simulink model "MBD_Triggerd_Subsystem"  (R2021b)
settings: Solver=FixedStepDiscrete  StartTime=0.0  StopTime=10.0  FixedStep=0.001  RelTol=1e-3
libraries: simulink x1
settings Model: Creator=waleed.elshemy  LastModifiedBy=waleed.elshemy
settings OptimizationCC: DefaultParameterBehavior=Inlined  UseDivisionForNetSlopeComputation=on  GainParamInheritBuiltInType=on  UseFloatMulNetSlope=on  InlineInvariantSignals=on  PassReuseOutputArgsAs=Individual arguments  ZeroExternalMemoryAtStartup=off  ZeroInternalMemoryAtStartup=off  NoFixptDivByZeroProtection=on  EfficientFloat2IntCast=on  LifeSpan=1  OptimizeBlockOrder=speed  DifferentSizesBufferReuse=on  EfficientTunableParamExpr=on
settings DebuggingCC: ParameterTunabilityLossMsg=error
settings HardwareCC: ProdLongLongMode=on
settings SFSimCC: MATLABDynamicMemAlloc=off
settings RTWCC: Description=Embedded Coder  SystemTargetFile=ert.tlc  TemplateMakefile=ert_default_tmf
settings CodeAppCC: ForceParamTrailComments=on  IgnoreCustomStorageClasses=off  OperatorAnnotations=on  SimulinkDataObjDesc=on  SFDataObjDesc=on  CustomSymbolStrGlobalVar=rt$N$M  CustomSymbolStrType=$N$M  CustomSymbolStrFcn=$N$M$F  CustomSymbolStrMacro=$N$M  InsertBlockDesc=on
settings ERTTargetCC: TargetLangStandard=C99 (ISO)  GenerateSampleERTMain=on  IncludeMdlTerminateFcn=off  CombineSignalStateStructs=on  CodeInterfacePackaging=Reusable function  SupportComplex=off  InlinedParameterPlacement=NonHierarchical  ERTCustomFileTemplate=example_file_process.tlc  ERTFilePackagingFormat=CompactWithDataFile

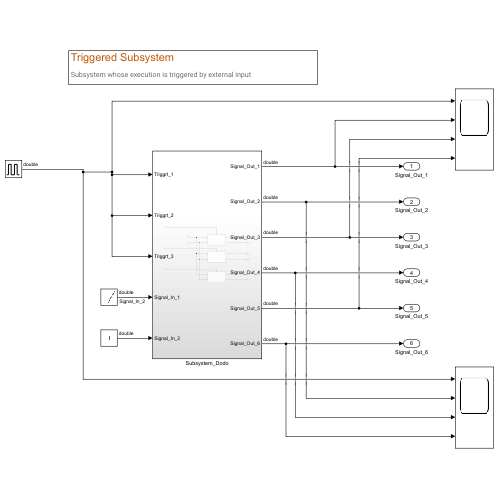
[thumbnail: Simulink's stored preview of the top-level diagram]
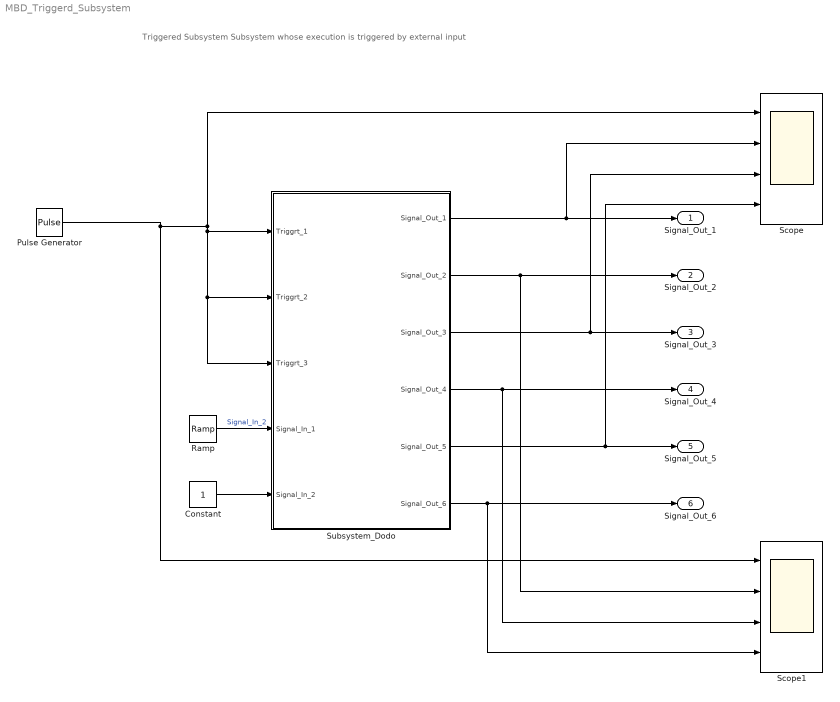
== system MBD_Triggerd_Subsystem ==
  note: Triggered Subsystem
      | Subsystem whose execution is triggered by external input
  Constant : Constant
  Pulse Generator : DiscretePulseGenerator  PulseType=Time based  Period=5  PulseWidth=50
  Ramp : simulink/Sources/Ramp  slope=1  start=0  InitialOutput=0
  Scope : Scope  NumInputPorts=4
  Scope1 : Scope  NumInputPorts=4
  Subsystem_Dodo : Subsystem
  Signal_Out_1 : Outport
  Signal_Out_2 : Outport  Port=2
  Signal_Out_3 : Outport  Port=3
  Signal_Out_4 : Outport  Port=4
  Signal_Out_5 : Outport  Port=5
  Signal_Out_6 : Outport  Port=6
  wires:
  Subsystem_Dodo/1(Signal_Out_1) -> Signal_Out_1/1, Scope/2
  Subsystem_Dodo/2(Signal_Out_2) -> Signal_Out_2/1, Scope1/2
  Subsystem_Dodo/3(Signal_Out_3) -> Signal_Out_3/1, Scope/3
  Subsystem_Dodo/4(Signal_Out_4) -> Signal_Out_4/1, Scope1/3
  Ramp/1 -> Subsystem_Dodo/4(Signal_In_1)  "Signal_In_2"
  Constant/1 -> Subsystem_Dodo/5(Signal_In_2)
  Pulse Generator/1 -> Scope1/1, Scope/1, Subsystem_Dodo/3(Triggrt_3), Subsystem_Dodo/2(Triggrt_2), Subsystem_Dodo/1(Triggrt_1)
  Subsystem_Dodo/6(Signal_Out_6) -> Signal_Out_6/1, Scope1/4
  Subsystem_Dodo/5(Signal_Out_5) -> Signal_Out_5/1, Scope/4

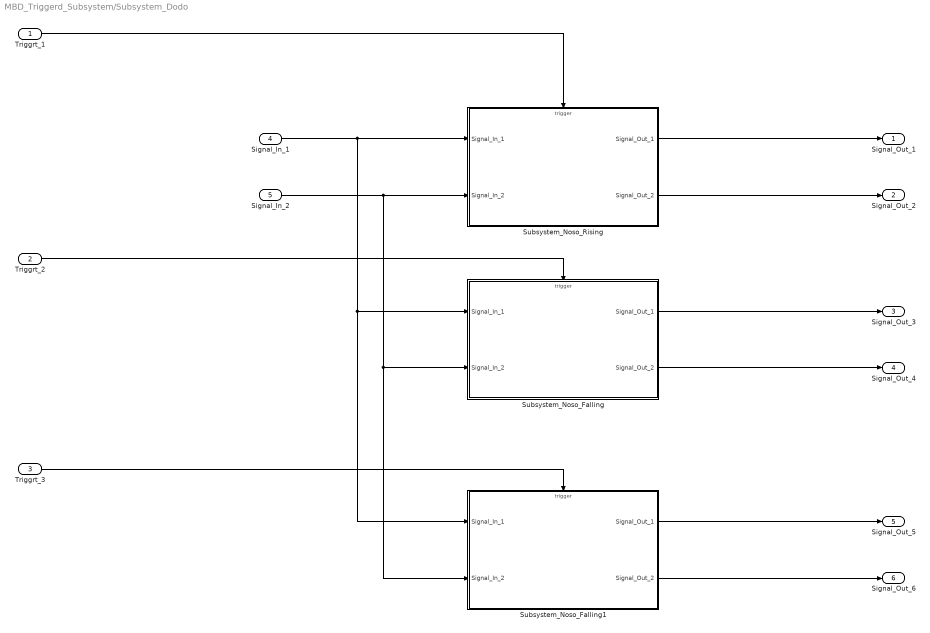
== system MBD_Triggerd_Subsystem/Subsystem_Dodo ==
  Triggrt_1 : Inport
  Triggrt_2 : Inport  Port=2
  Triggrt_3 : Inport  Port=3
  Signal_In_1 : Inport  Port=4
  Signal_In_2 : Inport  Port=5
  Subsystem_Noso_Falling : Subsystem  TreatAsAtomicUnit=on
      settings: RTWFileNameOpts=Use function name
  Subsystem_Noso_Falling1 : Subsystem  TreatAsAtomicUnit=on
      settings: RTWFileNameOpts=Use function name
  Subsystem_Noso_Rising : Subsystem  TreatAsAtomicUnit=on
  Signal_Out_1 : Outport
  Signal_Out_2 : Outport  Port=2
  Signal_Out_3 : Outport  Port=3
  Signal_Out_4 : Outport  Port=4
  Signal_Out_5 : Outport  Port=5
  Signal_Out_6 : Outport  Port=6
  wires:
  Subsystem_Noso_Rising/1(Signal_Out_1) -> Signal_Out_1/1
  Signal_In_2/1 -> Subsystem_Noso_Falling1/2(Signal_In_2), Subsystem_Noso_Falling/2(Signal_In_2), Subsystem_Noso_Rising/2(Signal_In_2)
  Subsystem_Noso_Rising/2(Signal_Out_2) -> Signal_Out_2/1
  Subsystem_Noso_Falling/1(Signal_Out_1) -> Signal_Out_3/1
  Subsystem_Noso_Falling/2(Signal_Out_2) -> Signal_Out_4/1
  Triggrt_2/1 -> Subsystem_Noso_Falling/Trigger
  Triggrt_1/1 -> Subsystem_Noso_Rising/Trigger
  Subsystem_Noso_Falling1/2(Signal_Out_2) -> Signal_Out_6/1
  Signal_In_1/1 -> Subsystem_Noso_Falling1/1(Signal_In_1), Subsystem_Noso_Falling/1(Signal_In_1), Subsystem_Noso_Rising/1(Signal_In_1)
  Subsystem_Noso_Falling1/1(Signal_Out_1) -> Signal_Out_5/1
  Triggrt_3/1 -> Subsystem_Noso_Falling1/Trigger

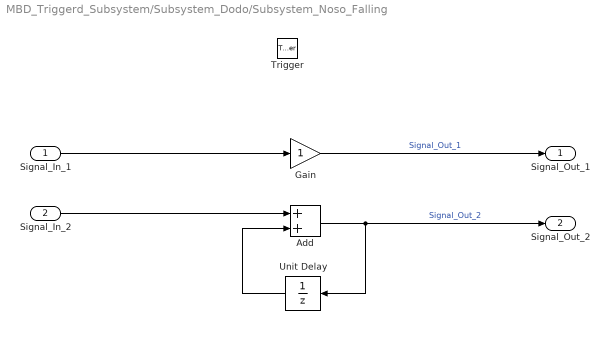
== system MBD_Triggerd_Subsystem/Subsystem_Dodo/Subsystem_Noso_Falling ==
  Signal_In_1 : Inport
  Signal_In_2 : Inport  Port=2
  Trigger : TriggerPort  TriggerType=falling  VariantControl=(inherit)  PortDimensions=1
  Add : Sum
  Gain : Gain
  Unit Delay : UnitDelay  SampleTime=-1  HasFrameUpgradeWarning=on
  Signal_Out_1 : Outport
  Signal_Out_2 : Outport  Port=2
  wires:
  Signal_In_1/1 -> Gain/1
  Unit Delay/1 -> Add/2
  Signal_In_2/1 -> Add/1
  Gain/1 -> Signal_Out_1/1  "Signal_Out_1"
  Add/1 -> Unit Delay/1, Signal_Out_2/1  "Signal_Out_2"

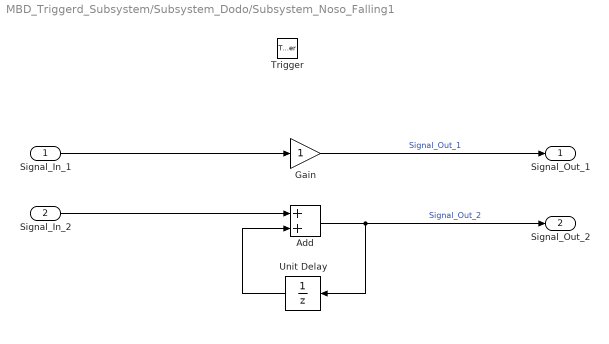
== system MBD_Triggerd_Subsystem/Subsystem_Dodo/Subsystem_Noso_Falling1 ==
  Signal_In_1 : Inport
  Signal_In_2 : Inport  Port=2
  Trigger : TriggerPort  TriggerType=either  VariantControl=(inherit)  PortDimensions=1
  Add : Sum
  Gain : Gain
  Unit Delay : UnitDelay  SampleTime=-1  HasFrameUpgradeWarning=on
  Signal_Out_1 : Outport
  Signal_Out_2 : Outport  Port=2
  wires:
  Signal_In_1/1 -> Gain/1
  Unit Delay/1 -> Add/2
  Signal_In_2/1 -> Add/1
  Gain/1 -> Signal_Out_1/1  "Signal_Out_1"
  Add/1 -> Unit Delay/1, Signal_Out_2/1  "Signal_Out_2"

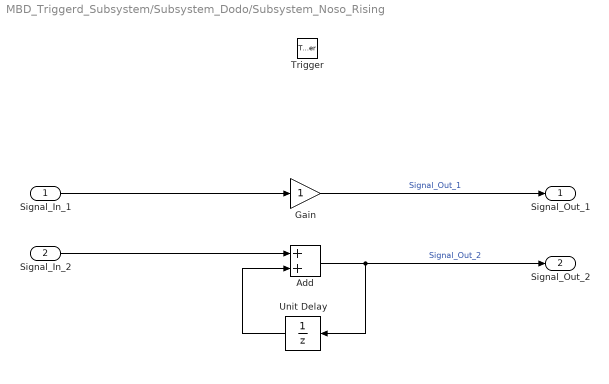
== system MBD_Triggerd_Subsystem/Subsystem_Dodo/Subsystem_Noso_Rising ==
  Signal_In_1 : Inport
  Signal_In_2 : Inport  Port=2
  Trigger : TriggerPort  VariantControl=(inherit)  PortDimensions=1
  Add : Sum
  Gain : Gain
  Unit Delay : UnitDelay  SampleTime=-1  HasFrameUpgradeWarning=on
  Signal_Out_1 : Outport
  Signal_Out_2 : Outport  Port=2
  wires:
  Add/1 -> Signal_Out_2/1, Unit Delay/1  "Signal_Out_2"
  Gain/1 -> Signal_Out_1/1  "Signal_Out_1"
  Signal_In_2/1 -> Add/1
  Unit Delay/1 -> Add/2
  Signal_In_1/1 -> Gain/1
